simulink model "dynamic_extension_closed_loop"  (R2015b)
settings: Solver=ode1  StartTime=0.0  StopTime=25  FixedStep=0.002  RelTol=1e-3
values from neighbouring files (symbols this model uses):
  K = place(A', C', p)'    [high_gain_pole_placement.m]    (also in tvlqr_feedback_trajectory.m = zeros(length(t), m, n); tvlqri_feedback_trajectory.m = zeros(length(t), m, n); weird_observer_pole_placement.m)
  lamb = [0  0  0  0  0; 0  0  0  0  0]    [dyn_ext_eps_static_meas.mat]    (also in extend_static_trajectory.m = repmat(lamb, samples, 1); high_gain_obs_test_meas_using_obs_for_contr.mat = [0 1.24633399283e-14 3.94751216865e-13 2.99125768707e-12 1.2; high_gain_obs_test_meas_using_obs_for_contr_2.mat = [0 0 0 0 0 0 0 0 0 0 0 0 ... (30000 elements, 6000x5)]; high_gain_obs_test_meas_using_obs_for_contr_3.mat = [0 0 0 0 0 0 0 0 0 0 0 0 ... (30000 elements, 6000x5)])
  phi = [0  0  0; 0  0  0]    [dyn_ext_eps_static_meas.mat]    (also in extend_static_trajectory.m = repmat(phi, samples, 1); high_gain_obs_test_meas_using_obs_for_contr.mat = [1.104382406e-14 3.36532550257e-09 2.6875311489e-08 9.054493; high_gain_obs_test_meas_using_obs_for_contr_2.mat = [0 0 0 0 0 0 0 0 0 0 0 0 ... (18000 elements, 6000x3)]; high_gain_obs_test_meas_using_obs_for_contr_3.mat = [0 0 0 0 0 0 0 0 0 0 0 0 ... (18000 elements, 6000x3)])
  vb = [3.51031402612 3.51031402612]    [dyn_ext_eps_static_meas.mat]    (also in extend_static_trajectory.m = repmat(vb, samples, 1); high_gain_obs_test_meas_using_obs_for_contr.mat = [3.03305943788 3.03299005654 3.03292056635 3.03285098117 3.0; high_gain_obs_test_meas_using_obs_for_contr_2.mat = [2.46662433384 2.46662437608 2.46662467016 2.46662546356 2.4; high_gain_obs_test_meas_using_obs_for_contr_3.mat = [2.46662433384 2.46662437608 2.46662467016 2.46662546356 2.4)
  vf = [3.51031402612 3.51031402612]    [dyn_ext_eps_static_meas.mat]    (also in extend_static_trajectory.m = repmat(vf, samples, 1); high_gain_obs_test_meas_using_obs_for_contr.mat = [3.03305943788 3.03312882088 3.03319832259 3.03326793896 3.0; high_gain_obs_test_meas_using_obs_for_contr_2.mat = [2.46662433384 2.46662437608 2.46662467016 2.46662546356 2.4; high_gain_obs_test_meas_using_obs_for_contr_3.mat = [2.46662433384 2.46662437608 2.46662467016 2.46662546356 2.4)
libraries: simulink_extras x6
settings Model: ExtModeTrigDuration=5000  Creator=robertph  LastModifiedBy=Robert
settings SolverCC: PositivePriorityOrder=on
settings RTWCC: SystemTargetFile=quarc_win64.tlc  TemplateMakefile=quarc_default_tmf  Description=QUARC Win64 Target
settings STFCustomTargetCC: GeneratePreprocessorConditionals=Use local settings  CPPClassGenCompliant=off
settings GRTTargetCC: ParMdlRefBuildCompliant=off  CompOptLevelCompliant=off  CombineOutputUpdateFcns=off  MatFileLogging=off  CPPClassGenCompliant=off  GRTInterface=on  UseToolchainInfoCompliant=off  ExtMode=on  ExtModeMexFile=quarc_comm

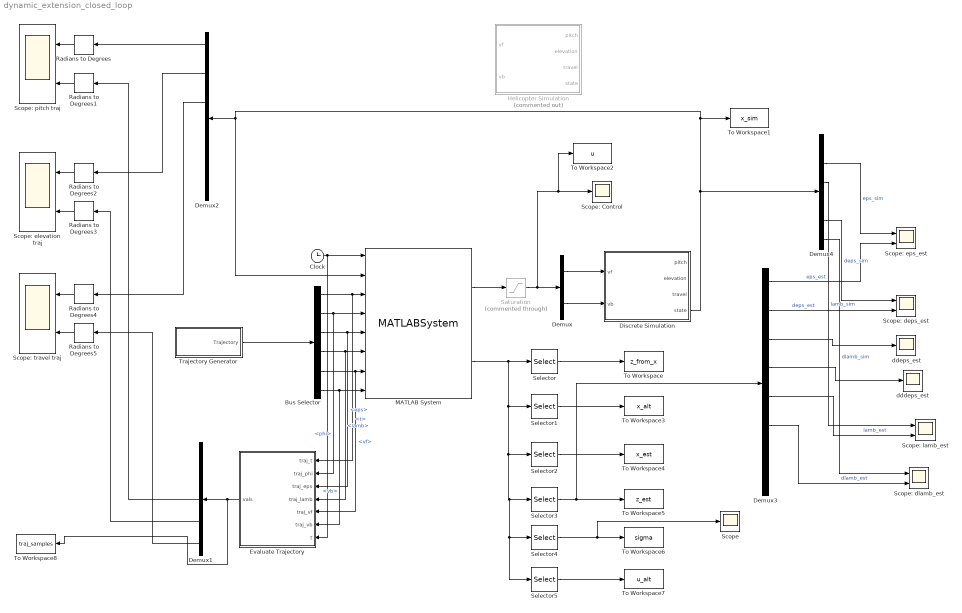
== system dynamic_extension_closed_loop ==
  Bus Selector : BusSelector  OutputSignals=t,phi,eps,lamb,vf,vb
  Clock : Clock
  Demux : Demux  Outputs=2
  Demux1 : Demux  Outputs=5
  Demux2 : Demux  Outputs=6
  Demux3 : Demux  Outputs=8
  Demux4 : Demux  Outputs=6
  Discrete Simulation : Subsystem  VariantControl=DiscreteSim  mask{ang0=[0, -8, 2], dang0=[0, 0, 0], h=0.002}
      mask prompts: ang0 "Pitch, Elevation, Travel (deg)"; dang0 "Angular velocities (deg/s)"; h "Sample time"
      mask DialogControl DescGroupVar Prompt: Helicopter Simulation
      mask DialogControl DescTextVar Prompt: Simulates the helicopter system based on the equations of motion specified in system_f.m
      mask DialogControl ParameterGroupVar Prompt: Initial values
  Evaluate Trajectory : MATLAB Function  TreatAsAtomicUnit=on
  Helicopter Simulation : Subsystem  Commented=on  VariantControl=BetterSim  mask{ang0=[0, -20, 0], dang0=[0, 0, 0], w0=[0, 0]}
      mask prompts: ang0 "Pitch, Elevation, Travel (deg)"; dang0 "Angular velocities (deg/s)"; w0 "Rotor velocities"
      mask DialogControl DescTextVar Prompt: Simulates the helicopter system based on the equations of motion specified in system_f.m
  MATLAB System : MATLABSystem  System=DynamicExtension  k_eps=[64 48 12 1]  k_lamb=[20 22 8 1]  a1=10  a2=30  b1=100  b2=0.1  K=K  x780=x780  z_est0=z_est0  x_est0=x_est0  step_width=0.002  smc=on  use_high_gain_observer=on  use_weird_observer=off  SimulateUsing=Code generation
      mask Type: DynamicExtension
      mask Display:
      | disp('DynamicExtension');
      | port_label('input',1,'Time');
      | port_label('input',2,'State');
      | port_label('input',3,'Traj Time');
      | port_label('input',4,'Traj Phi');
      | port_label('input',5,'Traj Eps');
      | port_label('input',6,'Traj Lamb');
      | port_label('input',7,'Traj Vf');
      | port_label('input',8,'Traj Vb');
      | port_label('output',1,'Control');
      | port_label('output',2,'Debug');
  Radians to Degrees{,1..5} (6 alike) : simulink_extras/Transformations/Radians to Degrees
  Saturation : Saturate  Commented=through  UpperLimit=5  LowerLimit=-5
  Scope : Scope
  Scope: Control : Scope
  Scope: deps_est : Scope  NumInputPorts=2
  Scope: dlamb_est : Scope  NumInputPorts=2
  Scope: elevation traj : Scope  NumInputPorts=2
  Scope: eps_est : Scope  NumInputPorts=2
  Scope: lamb_est : Scope  NumInputPorts=2
  Scope: pitch traj : Scope  NumInputPorts=2
  Scope: travel traj : Scope  NumInputPorts=2
  Selector : Selector  InputPortWidth=44  IndexOptions=Index vector (dialog)  Indices=[37,38,39,40,41,42,43,44]  OutputSizes=1
  Selector1 : Selector  InputPortWidth=44  IndexOptions=Index vector (dialog)  Indices=[1, 2, 3, 4, 5, 6, 7, 8]  OutputSizes=1
  Selector2 : Selector  InputPortWidth=44  IndexOptions=Index vector (dialog)  Indices=[9:16]  OutputSizes=1
  Selector3 : Selector  InputPortWidth=44  IndexOptions=Index vector (dialog)  Indices=[17:24]  OutputSizes=1
  Selector4 : Selector  InputPortWidth=44  IndexOptions=Index vector (dialog)  Indices=[25:26]  OutputSizes=1
  Selector5 : Selector  InputPortWidth=44  IndexOptions=Index vector (dialog)  Indices=[29:30]  OutputSizes=1
  To Workspace : ToWorkspace  VariableName=z_from_x  SaveFormat=Structure With Time  SampleTime=-1
  To Workspace1 : ToWorkspace  VariableName=x_sim  SaveFormat=Structure With Time  SampleTime=-1
  To Workspace2 : ToWorkspace  VariableName=u  SaveFormat=Structure With Time  SampleTime=-1
  To Workspace3 : ToWorkspace  VariableName=x_alt  SaveFormat=Structure With Time  SampleTime=-1
  To Workspace4 : ToWorkspace  VariableName=x_est  SaveFormat=Structure With Time  SampleTime=-1
  To Workspace5 : ToWorkspace  VariableName=z_est  SaveFormat=Structure With Time  SampleTime=-1
  To Workspace6 : ToWorkspace  VariableName=sigma  SaveFormat=Structure With Time  SampleTime=-1
  To Workspace7 : ToWorkspace  VariableName=u_alt  SaveFormat=Structure With Time  SampleTime=-1
  To Workspace8 : ToWorkspace  VariableName=traj_samples  SaveFormat=Structure With Time  SampleTime=-1
  Trajectory Generator : Subsystem
  dddeps_est : Scope
  ddeps_est : Scope
  wires:
  Demux/2 -> Discrete Simulation/2(vb)
  Demux/1 -> Discrete Simulation/1(vf)
  Clock/1 -> MATLAB System/1, Evaluate Trajectory/7(t)
  Bus Selector/1 -> Evaluate Trajectory/1(traj_t), MATLAB System/3  "<t>"
  Bus Selector/2 -> MATLAB System/4, Evaluate Trajectory/2(traj_phi)  "<phi>"
  Bus Selector/3 -> Evaluate Trajectory/3(traj_eps), MATLAB System/5  "<eps>"
  Bus Selector/4 -> Evaluate Trajectory/4(traj_lamb), MATLAB System/6  "<lamb>"
  Bus Selector/5 -> Evaluate Trajectory/5(traj_vf), MATLAB System/7  "<vf>"
  Bus Selector/6 -> Evaluate Trajectory/6(traj_vb), MATLAB System/8  "<vb>"
  Trajectory Generator/1(Trajectory) -> Bus Selector/1
  Evaluate Trajectory/1(vals) -> To Workspace8/1, Demux1/1
  Demux2/1 -> Radians to Degrees/1
  Demux2/2 -> Radians to Degrees2/1
  Demux2/3 -> Radians to Degrees4/1
  Radians to Degrees/1 -> Scope: pitch traj/1
  Radians to Degrees1/1 -> Scope: pitch traj/2
  Radians to Degrees2/1 -> Scope: elevation traj/1
  Radians to Degrees3/1 -> Scope: elevation traj/2
  Radians to Degrees4/1 -> Scope: travel traj/1
  Radians to Degrees5/1 -> Scope: travel traj/2
  Demux1/3 -> Radians to Degrees1/1
  Demux1/4 -> Radians to Degrees3/1
  Demux1/5 -> Radians to Degrees5/1
  MATLAB System/1 -> Saturation/1
  Discrete Simulation/4(state) -> MATLAB System/2, Demux2/1, To Workspace1/1, Demux4/1
  MATLAB System/2 -> Selector5/1, Selector4/1, Selector3/1, Selector2/1, Selector1/1, Selector/1
  Selector/1 -> To Workspace/1
  Saturation/1 -> To Workspace2/1, Scope: Control/1, Demux/1
  Selector1/1 -> To Workspace3/1
  Selector2/1 -> To Workspace4/1
  Selector3/1 -> Demux3/1, To Workspace5/1
  Selector4/1 -> Scope/1, To Workspace6/1
  Selector5/1 -> To Workspace7/1
  Demux4/2 -> Scope: eps_est/1  "eps_sim"
  Demux3/1 -> Scope: eps_est/2  "eps_est"
  Demux4/5 -> Scope: deps_est/1  "deps_sim"
  Demux3/2 -> Scope: deps_est/2  "deps_est"
  Demux3/3 -> ddeps_est/1
  Demux3/4 -> dddeps_est/1
  Demux3/5 -> Scope: lamb_est/2  "lamb_est"
  Demux4/3 -> Scope: lamb_est/1  "lamb_sim"
  Demux4/6 -> Scope: dlamb_est/1  "dlamb_sim"
  Demux3/6 -> Scope: dlamb_est/2  "dlamb_est"

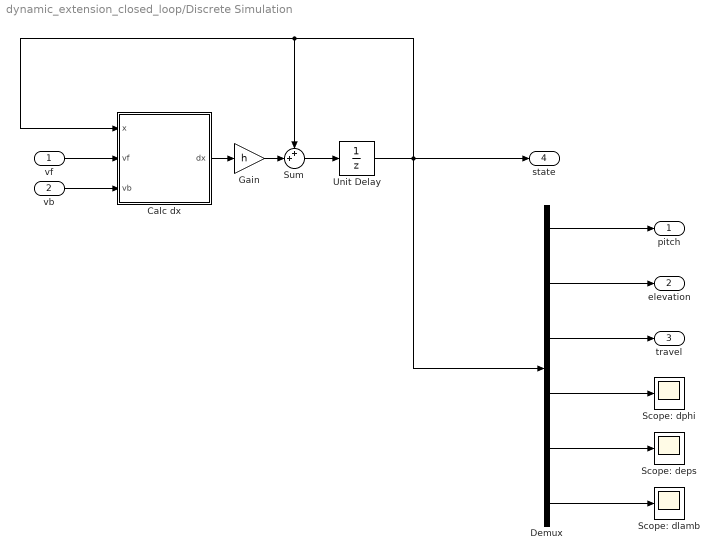
== system dynamic_extension_closed_loop/Discrete Simulation ==
  vf : Inport
  vb : Inport  Port=2
  Calc dx : MATLAB Function  TreatAsAtomicUnit=on
  Demux : Demux  Outputs=6
  Gain : Gain  Gain=h
  Scope: deps : Scope
  Scope: dlamb : Scope
  Scope: dphi : Scope
  Sum : Sum  Inputs=++|
  Unit Delay : UnitDelay  InitialCondition=[(ang0 / 180 * pi)'; (dang0 / 180 * pi)']  SampleTime=h
  pitch : Outport
  elevation : Outport  Port=2
  travel : Outport  Port=3
  state : Outport  Port=4  OutDataTypeStr=double  PortDimensions=6
  wires:
  vf/1 -> Calc dx/2(vf)
  vb/1 -> Calc dx/3(vb)
  Sum/1 -> Unit Delay/1
  Calc dx/1(dx) -> Gain/1
  Gain/1 -> Sum/2
  Demux/1 -> pitch/1
  Demux/2 -> elevation/1
  Demux/3 -> travel/1
  Demux/4 -> Scope: dphi/1
  Demux/5 -> Scope: deps/1
  Demux/6 -> Scope: dlamb/1
  Unit Delay/1 -> Sum/1, Calc dx/1(x), Demux/1, state/1

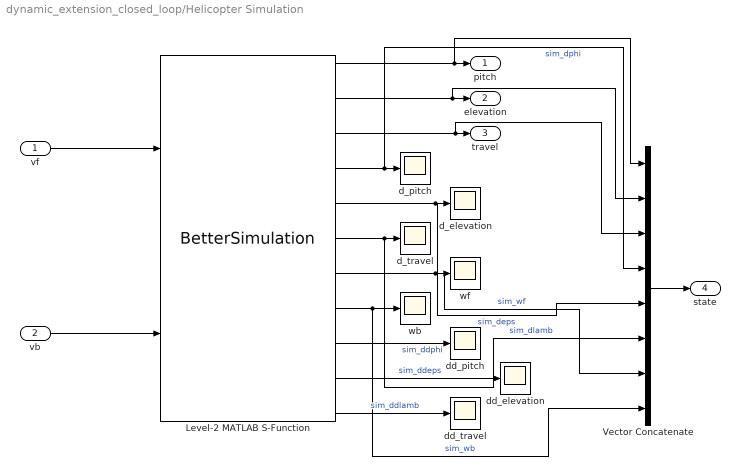
== system dynamic_extension_closed_loop/Helicopter Simulation ==
  vf : Inport
  vb : Inport  Port=2
  Level-2 MATLAB S-Function : M-S-Function  FunctionName=BetterSimulation  Parameters=ang0(1), ang0(2), ang0(3), dang0(1), dang0(2), dang0(3), w0(1), w0(2)
  Vector Concatenate : Concatenate  NumInputs=8
  d_elevation : Scope
  d_pitch : Scope
  d_travel : Scope
  dd_elevation : Scope
  dd_pitch : Scope
  dd_travel : Scope
  wb : Scope
  wf : Scope
  pitch : Outport
  elevation : Outport  Port=2
  travel : Outport  Port=3
  state : Outport  Port=4
  wires:
  vf/1 -> Level-2 MATLAB S-Function/1
  vb/1 -> Level-2 MATLAB S-Function/2
  Level-2 MATLAB S-Function/1 -> Vector Concatenate/1, pitch/1
  Level-2 MATLAB S-Function/3 -> Vector Concatenate/3, travel/1
  Level-2 MATLAB S-Function/2 -> Vector Concatenate/2, elevation/1
  Level-2 MATLAB S-Function/4 -> Vector Concatenate/4, d_pitch/1  "sim_dphi"
  Level-2 MATLAB S-Function/8 -> Vector Concatenate/8, wb/1  "sim_wb"
  Level-2 MATLAB S-Function/7 -> Vector Concatenate/7, wf/1  "sim_wf"
  Level-2 MATLAB S-Function/6 -> Vector Concatenate/6, d_travel/1  "sim_dlamb"
  Level-2 MATLAB S-Function/5 -> Vector Concatenate/5, d_elevation/1  "sim_deps"
  Level-2 MATLAB S-Function/10 -> dd_elevation/1  "sim_ddeps"
  Level-2 MATLAB S-Function/11 -> dd_travel/1  "sim_ddlamb"
  Level-2 MATLAB S-Function/9 -> dd_pitch/1  "sim_ddphi"
  Vector Concatenate/1 -> state/1

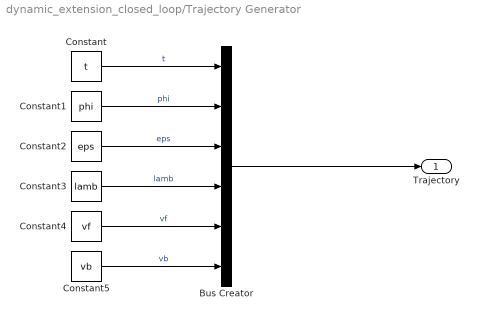
== system dynamic_extension_closed_loop/Trajectory Generator ==
  Bus Creator : BusCreator  Inputs=6
  Constant : Constant  Value=t
  Constant1 : Constant  Value=phi  VectorParams1D=off
  Constant2 : Constant  Value=eps  VectorParams1D=off
  Constant3 : Constant  Value=lamb  VectorParams1D=off
  Constant4 : Constant  Value=vf  VectorParams1D=off
  Constant5 : Constant  Value=vb  VectorParams1D=off
  Trajectory : Outport
  wires:
  Constant/1 -> Bus Creator/1  "t"
  Constant5/1 -> Bus Creator/6  "vb"
  Constant4/1 -> Bus Creator/5  "vf"
  Constant3/1 -> Bus Creator/4  "lamb"
  Constant2/1 -> Bus Creator/3  "eps"
  Constant1/1 -> Bus Creator/2  "phi"
  Bus Creator/1 -> Trajectory/1

== matlab function dynamic_extension_closed_loop/Evaluate Trajectory ==
  data: traj_t input; traj_phi input; traj_eps input; traj_lamb input; traj_vf input; traj_vb input; vals output; t input
function vals  = fcn(traj_t, traj_phi, traj_eps, traj_lamb, traj_vf, traj_vb, t)
traj = struct('t', traj_t, 'phi', traj_phi, 'eps', traj_eps, 'lamb', traj_lamb, 'vf', traj_vf, 'vb', traj_vb);
traj_eval = eval_trajectory(traj, t);

vals = zeros(5, 1);
vals(1) = traj_eval.vf(1);
vals(2) = traj_eval.vb(1);
vals(3) = traj_eval.phi(1);
vals(4) = traj_eval.eps(1);
vals(5) = traj_eval.lamb(1);

== matlab function dynamic_extension_closed_loop/Discrete Simulation/Calc dx ==
  data: x input; dx output; vf input; vb input
function dx = fcn(x, vf, vb)
%#codegen

dx = system_f(x, [vf; vb], true);
